simulink model "tableUsageExample"  (R2019b)
settings: Solver=VariableStepAuto  StartTime=0.0  StopTime=10.0  RelTol=1e-3
undefined symbols (not defined in the file or in its folder): datMotor
settings Model: Creator=swami  LastModifiedBy=swami

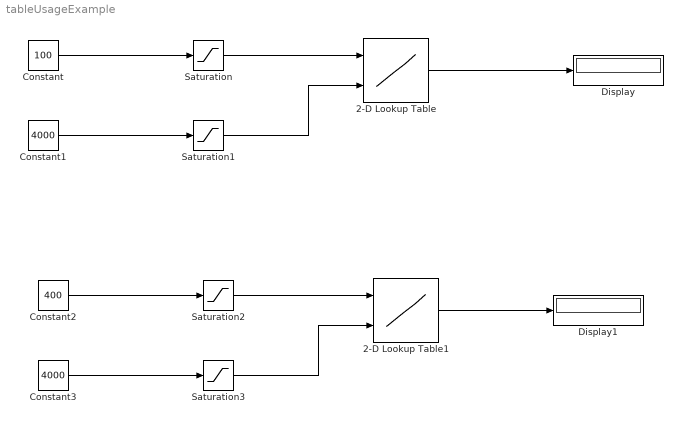
== system tableUsageExample ==
  2-D Lookup Table : Lookup_n-D  BreakpointsForDimension1=datMotor.eta_torque  BreakpointsForDimension2=datMotor.eta_speed  Table=datMotor.eta_val  InternalRulePriority=Speed  RndMeth=Simplest  InputSameDT=on
  2-D Lookup Table1 : Lookup_n-D  BreakpointsForDimension1=datMotor.vbus  BreakpointsForDimension2=datMotor.rpm  Table=datMotor.maxtorque  InternalRulePriority=Speed  RndMeth=Simplest  InputSameDT=on
  Constant : Constant  Value=100
  Constant1 : Constant  Value=4000
  Constant2 : Constant  Value=400
  Constant3 : Constant  Value=4000
  Display : Display
  Display1 : Display
  Saturation : Saturate  UpperLimit=325  LowerLimit=0
  Saturation1 : Saturate  UpperLimit=10000  LowerLimit=0
  Saturation2 : Saturate  UpperLimit=450  LowerLimit=250
  Saturation3 : Saturate  UpperLimit=10000  LowerLimit=0
  wires:
  Constant/1 -> Saturation/1
  Saturation/1 -> 2-D Lookup Table/1
  Constant1/1 -> Saturation1/1
  Saturation1/1 -> 2-D Lookup Table/2
  2-D Lookup Table/1 -> Display/1
  Saturation3/1 -> 2-D Lookup Table1/2
  Constant3/1 -> Saturation3/1
  Saturation2/1 -> 2-D Lookup Table1/1
  Constant2/1 -> Saturation2/1
  2-D Lookup Table1/1 -> Display1/1
